simulink model "req18"  (R2019a)
settings: Solver=FixedStepAuto  StartTime=0.0  StopTime=100  RelTol=1e-3
settings Model: Creator=e40014285  LastModifiedBy=e40014285
settings ConfigComp: CovScope=ReferencedModels  CovHTMLOptions=-sRT=1 -sVT=0 -aTS=1 -bRG=1 -bTC=1 -hTR=0 -nFC=0 -nFD=1 -scm=1 -bcm=1 -xEv=0 -xEM=0  CovHtmlReporting=on  CovCumulativeReport=on  DVMaxProcessTime=6000  DVModelCoverageObjectives=EnhancedMCDC  DVTestSuiteOptimization=Auto  DVDetectOutOfBounds=on  DVReportPDFFormat=on  DVRebuildModelRepresentation=Always

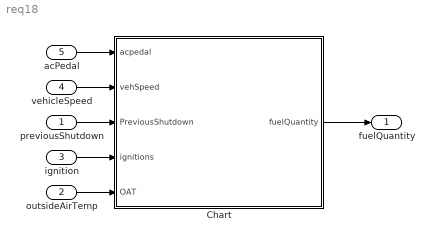
== system req18 ==
  previousShutdown : Inport
  outsideAirTemp : Inport  Port=2
  ignition : Inport  Port=3
  vehicleSpeed : Inport  Port=4
  acPedal : Inport  Port=5
  Chart : Stateflow chart  BlockKeywords=__PRM__SERIALIZED__DATA__:Stateflow Chart,Stateflow Diagram  TreatAsAtomicUnit=on
  fuelQuantity : Outport
  wires:
  Chart/1(fuelQuantity) -> fuelQuantity/1
  previousShutdown/1 -> Chart/3(PreviousShutdown)
  outsideAirTemp/1 -> Chart/5(OAT)
  ignition/1 -> Chart/4(ignitions)
  vehicleSpeed/1 -> Chart/2(vehSpeed)
  acPedal/1 -> Chart/1(acpedal)

== stateflow chart req18/Chart ==
  state total
    state vehstate [parallel]
      settings: executionOrder=1
      state running
        vehState=2;
      state init
      state off
        vehState=0;
      state on
        vehState=1;
      (default) -> init : {vehState=0;}
      init -> total.vehstate.running [order 3] : [ignitions==1&&vehSpeed>0]
      total.vehstate.running -> init : [~(ignitions==1&&vehSpeed>0)]
      init -> off [order 1] : [ignitions==0&&vehSpeed==0]
      off -> init : [~(ignitions==0&&vehSpeed==0)]
      on -> init : [~(ignitions==1&&vehSpeed==0)]
      init -> on [order 2] : [ignitions==1&&vehSpeed==0]
    state fuelQuantity [parallel]
      settings: executionOrder=2
      state running
        fuelQuantity=acpedal;
      state default
      state coldStart
        fuelQuantity=80;
      state warmStart
        fuelQuantity=50;
      state hotstart
        fuelQuantity=50;
      (default) -> default
      default -> total.fuelQuantity.running [order 4] : [vehState==2]
      total.fuelQuantity.running -> default : [vehState~=2]
      default -> coldStart [order 1] : [PreviousShutdown>5&&OAT<20&&vehState==0]
      coldStart -> default : [~(PreviousShutdown>5&&OAT<20&&vehState==0)]
      default -> warmStart [order 3] : [PreviousShutdown<=5 && OAT<20 && vehState==1]
      warmStart -> default : [~(PreviousShutdown<=5 && OAT<20 &&vehState==1)]
      default -> hotstart [order 2] : [OAT>20 && (vehState==1||vehState==0)]
      hotstart -> default : [~(OAT>20 && (vehState==1||vehState==0))]
  (default) -> total
  data: acpedal input; vehSpeed input; PreviousShutdown input; ignitions input; vehState local; fuelQuantity output; OAT input
